simulink model "GMCLIB_DecouplingPMSM_BAM"  (Simulink 9.3)
settings: Solver=VariableStepAuto  StartTime=0.0  StopTime=10.0  RelTol=1e-3
settings Model: Creator=nxa18952  LastModifiedBy=nxa18952
settings DataIOCC: SaveFormat=Dataset  SignalLoggingSaveFormat=Dataset  ReturnWorkspaceOutputs=on
settings OptimizationCC: LifeSpan=auto
settings DebuggingCC: UnderspecifiedInitializationDetection=Simplified  MergeDetectMultiDrivingBlocksExec=error  FcnCallInpInsideContextMsg=error  SFUnexpectedBacktrackingDiag=error  SFNoUnconditionalDefaultTransitionDiag=error  SFExecutionAtInitializationDiag=warning  ArithmeticOperatorsInVariantConditions=error
settings HardwareCC: ProdBitPerPointer=64  ProdBitPerSizeT=64  ProdBitPerPtrDiffT=64  ProdLargestAtomicFloat=Float  ProdIntDivRoundTo=Zero  ProdEndianess=LittleEndian  ProdWordSize=64  ProdHWDeviceType=Intel->x86-64 (Windows64)
settings ModelReferenceCC: PropagateSignalLabelsOutOfModel=on
settings SFSimCC: SimUseLocalCustomCode=on
settings RTWCC: RTWUseLocalCustomCode=on
settings CodeAppCC: StateflowObjectComments=off
settings GRTTargetCC: TargetLangStandard=C99 (ISO)  CombineOutputUpdateFcns=on  GRTInterface=off
settings ConfigComp: CovMetricSettings=dwe  CovHtmlReporting=off  CovSaveCumulativeToWorkspaceVar=off  CovSaveSingleToWorkspaceVar=off  CovExternalEMLEnable=on

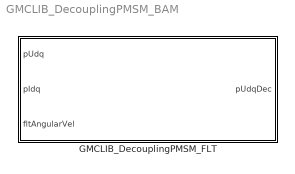
== system GMCLIB_DecouplingPMSM_BAM ==
  GMCLIB_DecouplingPMSM_FLT : Subsystem  TreatAsAtomicUnit=on  mask(GMCLIB_DecouplingPMSM_FLT){showStates=Hide (faster execution), fltLD=0, fltLQ=0}
      mask prompts: showStates "Show internal states"; fltLD "fltLD (D component of motor inductance [H])"; fltLQ "fltLQ (Q component of motor inductance [H])"
      mask help: Decoupling of d and q axis of PMSM model in single precision floating-point implementation. Refer to the AMMCLIB User's Guide for further details.
      mask init:
      | if ~evalin('base','exist(''tS8'',''var'')')
      |   if (2 ~= exist('SWLIBS_Typedefs.mat','file'))
      |       error('File SWLIBS_Typedefs.mat is not on the Matlab path. Please add the AMMCLIB "bam" folder in the Matlab Search Path.');
      |   else
      |       evalin('base', 'load(''SWLIBS_Typedefs.mat'')');
      |   end
      | end
      | if showStates == 1
      |     % hidden state variables
      |     if strcmp(get_param([gcb '/fltLD'], 'BlockType'), 'Inport')
      |         posblk = get_param(gcb, 'Position');
      | 
      |         pos = get_param(    [gcb, '/fltLD'], 'Position');
      |         orient = get_param( [gcb, '/fltLD'], 'Orientation');
      |         delete_block(       [gcb, '/fltLD']);
      |         add_block('built-in/Ground', [gcb, '/fltLD'], 'Position', pos, 'Orientation', orient);
      | 
      |         pos = get_param(    [gcb, '/fltLQ'], 'Position');
      |         orient = get_param( [gcb, '/fltLQ'], 'Orientation');
      |         delete_block(       [gcb, '/fltLQ']);
      |         add_block('built-in/Ground', [gcb, '/fltLQ'], 'Position', pos, 'Orientation', orient);
      | 
      | 
      | 
      |         set_param([gcb '/pUdq'], 'Port', '1');
      |         set_param([gcb '/pIdq'], 'Port', '2');
      |         set_param([gcb '/fltAngularVel'], 'Port', '3');
      | 
      |         set_param([gcb '/pUdqDec'], 'Port', '1');
      | 
      |         set_param(gcb,'MaskEnables',{'on','on','on'});
      | 
      |         if (posblk(4) - posblk(2)) > 100
      |           height = 100;
      |           set_param(gcb,'Position',[posblk(1), posblk(2), posblk(3), posblk(2)+height])
      |         end
      |     end
      | else
      |     % shown state variables
      |     if strcmp(get_param([gcb '/fltLD'], 'BlockType'), 'Ground')
      |         posblk = get_param(gcb, 'Position');
      | 
      |         pos = get_param(    [gcb, '/fltLD'], 'Position');
      |         orient = get_param( [gcb, '/fltLD'], 'Orientation');
      |         delete_block(       [gcb, '/fltLD']);
      |         add_block('built-in/Inport', [gcb, '/fltLD'], 'Position', pos, 'Orientation', orient, 'OutDataTypeStr', 'single');
      | 
      |         pos = get_param(    [gcb, '/fltLQ'], 'Position');
      |         orient = get_param( [gcb, '/fltLQ'], 'Orientation');
      |         delete_block(       [gcb, '/fltLQ']);
      |         add_block('built-in/Inport', [gcb, '/fltLQ'], 'Position', pos, 'Orientation', orient, 'OutDataTypeStr', 'single');
      | 
      | 
      | 
      |         set_param([gcb '/pUdq'], 'Port', '1');
      |         set_param([gcb '/pIdq'], 'Port', '2');
      |         set_param([gcb '/fltAngularVel'], 'Port', '3');
      |         set_param([gcb '/fltLD'], 'Port', '4');
      |         set_param([gcb '/fltLQ'], 'Port', '5');
      | 
      |         set_param([gcb '/pUdqDec'], 'Port', '1');
      | 
      |         set_param(gcb,'MaskEnables',{'on','off','off'});
      | 
      |         if (posblk(4) - posblk(2)) < 150
      |           height = 150;
      |           set_param(gcb,'Position',[posblk(1), posblk(2), posblk(3), posblk(2)+height])
      |         end
      |     end
      | end
      settings: RTWSystemCode=Inline
      mask TypeOptions showStates: Hide (faster execution) | Show (allows debugging; connect feedback loops manually)
      mask Callback showStates:
      | maskStr = get_param(gcb,'showStates');
      | if strcmp(maskStr,'Hide (faster execution)'),
      |     set_param(gcb,'MaskEnables',{'on','on','on'});
      | else
      |     set_param(gcb,'MaskEnables',{'on','off','off'});
      | end
      mask Display:
      | color('black');
      | pos = get_param(gcb, 'Position');
      | width = pos(3) - pos(1);
      | height = pos(4) - pos(2);
      | tX=width/2;
      | tY=height - 8;
      | color('black');
      | text(tX,tY, 'GMCLIB_DecouplingPMSM_FLT', 'horizontalAlignment', 'center');
      | if showStates == 2
      |   color('red');
      |   text(tX,tY - 20, ['debugging mode' char(13) char(10) '(limited performance)'], 'horizontalAlignment', 'center');
      | end

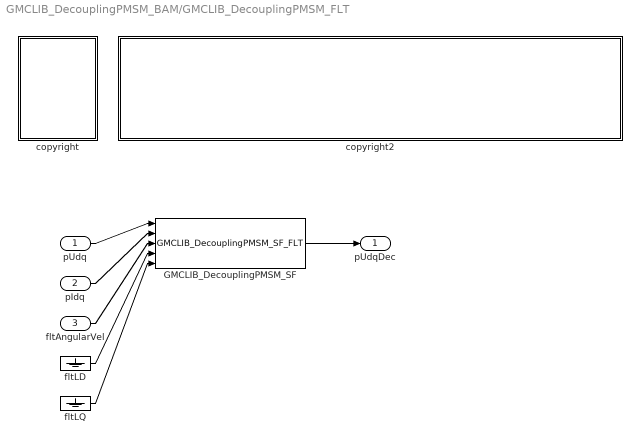
== system GMCLIB_DecouplingPMSM_BAM/GMCLIB_DecouplingPMSM_FLT ==
  pUdq : Inport  OutDataTypeStr=Bus: SWLIBS_2Syst_FLT  BusOutputAsStruct=on
  pIdq : Inport  Port=2  OutDataTypeStr=Bus: SWLIBS_2Syst_FLT  BusOutputAsStruct=on
  fltAngularVel : Inport  Port=3  OutDataTypeStr=single
  GMCLIB_DecouplingPMSM_SF : S-Function  FunctionName=GMCLIB_DecouplingPMSM_SF_FLT  Parameters=showStates,fltLD,fltLQ  SFunctionDeploymentMode=off  EnableBusSupport=off
  copyright : Subsystem
      mask Display: text(10,90,'FILE:');text(10,75,'DESRIPTION:');text(10,60,'COPYRIGHT:');text(10,45,'VERSION:');text(10,30,'DATE:')
  copyright2 : Subsystem
      mask Display: text(10,90,'GMCLIB_DecouplingPMSM_BAM_FLT.mdl');text(10,75,'Decoupling of d and q axis of PMSM model.');text(10,60,'NXP 2020');text(10,45,'1.0');text(10,30,'24-Mar-2020');
  fltLD : Ground
  fltLQ : Ground
  pUdqDec : Outport
  wires:
  pUdq/1 -> GMCLIB_DecouplingPMSM_SF/1
  pIdq/1 -> GMCLIB_DecouplingPMSM_SF/2
  fltAngularVel/1 -> GMCLIB_DecouplingPMSM_SF/3
  fltLD/1 -> GMCLIB_DecouplingPMSM_SF/4
  fltLQ/1 -> GMCLIB_DecouplingPMSM_SF/5
  GMCLIB_DecouplingPMSM_SF/1 -> pUdqDec/1

== system GMCLIB_DecouplingPMSM_BAM/GMCLIB_DecouplingPMSM_FLT/copyright ==

== system GMCLIB_DecouplingPMSM_BAM/GMCLIB_DecouplingPMSM_FLT/copyright2 ==
